simulink model "Ball_and_Plate_MicroLabBox"  (R2019b)
settings: Solver=ode1  StartTime=0.0  StopTime=Inf  FixedStep=0.001  RelTol=1e-3
PostLoadFcn:
  | , if any(exist('dsrtsu_mdlpostloadfcn', 'file') ~= 0), dsrtsu_mdlpostloadfcn('Execute', bdroot); end,
InitFcn:
  | , if any(exist('rtifpga_mdlclblib', 'file') ~= 0), rtifpga_mdlclblib('Init', bdroot); end,
undefined symbols (not defined in the file or in its folder): denc_mi, denco12_dis_des, denF, g, K, Kcam_x, Kcam_y, numc_mi, numco12_dis_des, numF, Ts_Outer
libraries: rtiemclib x6, rti1202lib_dac_class1 x3, rtiethernetlib x3, simulink x1
(part 2 of 2)

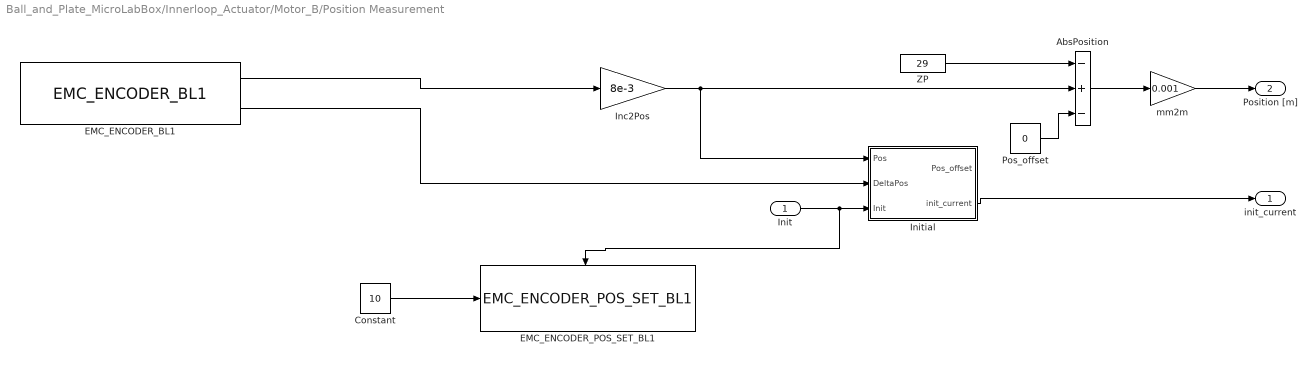
== system Ball_and_Plate_MicroLabBox/Innerloop_Actuator/Motor_B/Position Measurement ==
  Init : Inport
  AbsPosition : Sum  Inputs=-+-  SaturateOnIntegerOverflow=on
  Constant : Constant  Value=10
  EMC_ENCODER_BL1 : rtiemclib/EMC_ENCODER_BL1  DSProperties=struct('RTI',struct('Version',uint32(2),'BlockType',struct('isSLSource',uint8(1),'isSLSink',uint8(0),'isHWSource',uint8(1),'isHWSink',uint8(0),'isSetup',uint8(0),'isInline',uint8(1),'isNonInline',uint8(0),'isInterrupt',uint8(0),'isChannelwise',uint8(1)),'IOBoardType','DSEMC','UnitType','ENCODER','Identifier','ENCODER','DialogType','ML','BlockSet','RTIEMC','SlaveProcessor','NONE'))  RTIBlockInterface=struct('OutputPortsWidth',int32([1 1 1]),'OutputPortsActive',int32([1 1 0]),'OutputPortsName',{{'Position','Speed',['Index Detected']}},'OutputPortsDataType',{{'SS_DOUBLE','SS_DOUBLE','SS_BOOLEAN'}},'InitLevel',3,'IconTransparency','on','BlockDisplay',{{['EMC Encoder\nUnit: 2\nDIO class: 2\nPort: 1\nChannel: 3'],'center'}},'DialogFcn','rtiemcencodergui','BlockName',struct('Token',{{'EMC_ENCODER_BL1'}}))  RTIBlockParameters=struct('UnitNo',{{2,'OFF',[1 6]}},'DioClassNo',{{2,'OFF',[1 2]}},'PortNo',{{1,'OFF',[1 1]}},'ChannelNo',{{3,'OFF',[1 11]}},'HwSignalPin',{{['DIO1 ch1'],'OFF',[]}},'HwRefPin',{{'GND','OFF',[]}},'EnablePosMeasurement',{{1,'OFF',[0 1]}},'IndexSetMode',{{1,'OFF',[1 3]}},'EnableMinSpeed',{{0,'OFF',[0 1]}},'NumOfLines',{{'1024','OFF',[1 2097152]}},'InitAngleValue',{{'60','OFF',[0 359.99999]}},'IndexAngleValue',{{'0','OFF',[0 359.99999]}},'MinSpeedAngleValue',{{'45','OFF',[0.05 10000]}},'MinPosValue',{{'0','OFF',[-2097152 2097150.75]}},'MaxPosValue',{{'10000','OFF',[-2097151 2097151.75]}},'InitPosValue',{{'0','OFF',[-2097152 2097151.75]}},'IndexPosValue',{{'7500','OFF',[-2097152 2097151.75]}},'MinSpeedPosValue',{{'100','OFF',[1 1000000]}},'IndexGateMode',{{0,'OFF',[0 1]}},'EnableNoiseFilter',{{0,'OFF',[0 1]}},'FilterInterval',{{'0','OFF',[0 0.01]}},'IndexDetectedOutPortMode',{{0,'OFF',[0 1]}},'BuildCheckAngleMeasurement',{{0,'OFF',[0 1]}},'BuildCheckAngleIndexMode',{{0,'OFF',[0 1]}},'BuildCheckPosIndexMode',{{0,'OFF',[0 1]}},'BuildCheckAngleMinSpeed',{{0,'OFF',[0 1]}},'BuildCheckPosMinSpeed',{{0,'OFF',[0 1]}},'TLCFileName',{{'rtiemcencoder','OFF',[]}})  RTISFcnParameters=struct('UnitNo','int32','DioClassNo','int32','PortNo','int32','ChannelNo','int32','EnablePosMeasurement','int32','IndexSetMode','int32','IndexDetectedOutPortMode','int32','EnableMinSpeed','int32','NumOfLines','uint32','InitAngleValue','double','IndexAngleValue','double','MinSpeedAngleValue','double','MinPosValue','double','MaxPosValue','double','InitPosValue','double','IndexPosValue','double','MinSpeedPosValue','double','IndexGateMode','int32','EnableNoiseFilter','int32','FilterInterval','double','TLCFileName','char')  RTIBlockParaDefault=struct('UnitNo',1,'DioClassNo',1,'PortNo',1,'ChannelNo',1,'HwSignalPin',['DIO1 ch1'],'HwRefPin','GND','EnablePosMeasurement',0,'IndexSetMode',1,'EnableMinSpeed',0,'NumOfLines',1024,'InitAngleValue',60,'IndexAngleValue',0,'MinSpeedAngleValue',45,'MinPosValue',0,'MaxPosValue',1023.75,'InitPosValue',0,'IndexPosValue',0,'MinSpeedPosValue',100,'IndexGateMode',0,'EnableNoiseFilter',0,'FilterInterval',0,'IndexDetectedOutPortMode',0,'BuildCheckAngleMeasurement',1,'BuildCheckAngleIndexMode',0,'BuildCheckPosIndexMode',0,'BuildCheckAngleMinSpeed',0,'BuildCheckPosMinSpeed',0,'TLCFileName','rtiemcencoder')
      settings: SourceProductName=dSPACE RTI Electric Motor Control Blockset
  EMC_ENCODER_POS_SET_BL1 : rtiemclib/EMC_ENCODER_POS_SET_BL1  DSProperties=struct('RTI',struct('Version',uint32(1),'BlockType',struct('isSLSource',uint8(0),'isSLSink',uint8(1),'isHWSource',uint8(0),'isHWSink',uint8(1),'isSetup',uint8(0),'isInline',uint8(1),'isNonInline',uint8(0),'isInterrupt',uint8(0),'isChannelwise',uint8(1)),'IOBoardType','DSEMC','UnitType','ENCODER','Identifier','ENCODERPOSSET','DialogType','ML','BlockSet','RTIEMC','SlaveProcessor','NONE'))  RTIBlockInterface=struct('InputPortsWidth',int32(1),'InputPortsActive',1,'InputPortsDataType',{{'SS_DOUBLE'}},'InputPortsName',{{'Position'}},'TriggerPort',{{'rising'}},'InitLevel',3,'IconTransparency','on','BlockDisplay',{{['EMC Encoder Position Set\nUnit: 2\nDIO class: 2\nPort: 1\nChannel: 3'],'center'}},'DialogFcn','rtiemcencoderpossetgui','BlockName',struct('Token',{{'EMC_ENCODER_POS_SET_BL1'}}))  RTIBlockParameters=struct('EncoderIdIndex',{{3,'OFF',[1 4]}},'UnitNo',{{2,'OFF',[]}},'DioClassNo',{{2,'OFF',[]}},'PortNo',{{1,'OFF',[]}},'ChannelNo',{{3,'OFF',[]}},'EnablePosMeasurement',{{1,'OFF',[]}},'NumOfLines',{{1024,'OFF',[]}},'TLCFileName',{{'rtiemcencoderposset','OFF',[]}})  RTISFcnParameters=struct('EncoderIdIndex','int32','UnitNo','int32','DioClassNo','int32','PortNo','int32','ChannelNo','int32','EnablePosMeasurement','int32','NumOfLines','int32','TLCFileName','char')  RTIBlockParaDefault=struct('EncoderIdIndex',1,'UnitNo',-1,'DioClassNo',-1,'PortNo',-1,'ChannelNo',-1,'EnablePosMeasurement',0,'NumOfLines',1024,'TLCFileName','rtiemcencoderposset')
      settings: SourceProductName=dSPACE RTI Electric Motor Control Blockset
  Inc2Pos : Gain  Gain=8e-3  SaturateOnIntegerOverflow=on  OutDataTypeStr=Inherit: Same as input  ParamDataTypeStr=Inherit: Same as input
  Initial : Subsystem
  Pos_offset : Constant  Value=0
  ZP : Constant  Value=29
  mm2m : Gain  Gain=0.001
  init_current : Outport  VectorParamsAs1DForOutWhenUnconnected=off
  Position [m] : Outport  Port=2  VectorParamsAs1DForOutWhenUnconnected=off
  wires:
  AbsPosition/1 -> mm2m/1
  Inc2Pos/1 -> Initial/1(Pos), AbsPosition/2
  Initial/2(init_current) -> init_current/1
  mm2m/1 -> Position [m]/1
  EMC_ENCODER_BL1/2 -> Initial/2(DeltaPos)
  ZP/1 -> AbsPosition/1
  Init/1 -> EMC_ENCODER_POS_SET_BL1/Trigger, Initial/3(Init)
  Constant/1 -> EMC_ENCODER_POS_SET_BL1/1
  Pos_offset/1 -> AbsPosition/3
  EMC_ENCODER_BL1/1 -> Inc2Pos/1

== system Ball_and_Plate_MicroLabBox/Innerloop_Actuator/Motor_C/Outputs to Amplifier ==
  Motor current [A] : Inport
  Current2V : Gain  Gain=10/3  SaturateOnIntegerOverflow=on  OutDataTypeStr=Inherit: Same as input  ParamDataTypeStr=Inherit: Same as input
  DAC_CLASS1_BL1 : rti1202lib_dac_class1/DAC_CLASS1_BL1  DSProperties=struct('RTI',struct('Version',uint32(2),'BlockType',struct('isSLSource',uint8(0),'isSLSink',uint8(1),'isHWSource',uint8(0),'isHWSink',uint8(1),'isSetup',uint8(0),'isInline',uint8(1),'isNonInline',uint8(0),'isInterrupt',uint8(0),'isChannelwise',uint8(1)),'IOBoardType',{{'DS120X','STD','DACC1'}},'UnitType','DAC','Identifier','DAC','DialogType','ML','BlockSet','NONE','SlaveProcessor','NONE'))  RTIBlockInterface=struct('InputPortsActive',1,'InputPortsWidth',int32(1),'InputPortsDataType',{{'SS_DOUBLE'}},'InputPortsName',{{['DAC 3']}},'DialogFcn','rti120xstddacc1dacgui','InitLevel',3,'IconTransparency','on','BlockDisplay',{{['DAC CL1\nChannel: 3'],'center'}},'BlockName',struct('Token',{{'DAC_CLASS1_BL1'}}))  RTIBlockParameters=struct('ChannelNo',{{3,'OFF',[]}},'ChannelNumOf',{{1,'OFF',[]}},'InitialValue1',{{'0','OFF',[-10 10]}},'InitialValue2',{{'0','OFF',[-10 10]}},'InitialValue3',{{'0','OFF',[-10 10]}},'InitialValue4',{{'0','OFF',[-10 10]}},'InitialValue5',{{'0','OFF',[-10 10]}},'InitialValue6',{{'0','OFF',[-10 10]}},'InitialValue7',{{'0','OFF',[-10 10]}},'InitialValue8',{{'0','OFF',[-10 10]}},'InitialValue9',{{'0','OFF',[-10 10]}},'InitialValue10',{{'0','OFF',[-10 10]}},'InitialValue11',{{'0','OFF',[-10 10]}},'InitialValue12',{{'0','OFF',[-10 10]}},'InitialValue13',{{'0','OFF',[-10 10]}},'InitialValue14',{{'0','OFF',[-10 10]}},'InitialValue15',{{'0','OFF',[-10 10]}},'InitialValue16',{{'0','OFF',[-10 10]}},'OutputMode',{{ones(1,16),'OFF',[1 2]}},'TermValue1',{{'0','OFF',[-10 10]}},'TermValue2',{{'0','OFF',[-10 10]}},'TermValue3',{{'0','OFF',[-10 10]}},'TermValue4',{{'0','OFF',[-10 10]}},'TermValue5',{{'0','OFF',[-10 10]}},'TermValue6',{{'0','OFF',[-10 10]}},'TermValue7',{{'0','OFF',[-10 10]}},'TermValue8',{{'0','OFF',[-10 10]}},'TermValue9',{{'0','OFF',[-10 10]}},'TermValue10',{{'0','OFF',[-10 10]}},'TermValue11',{{'0','OFF',[-10 10]}},'TermValue12',{{'0','OFF',[-10 10]}},'TermValue13',{{'0','OFF',[-10 10]}},'TermValue14',{{'0','OFF',[-10 10]}},'TermValue15',{{'0','OFF',[-10 10]}},'TermValue16',{{'0','OFF',[-10 10]}},'EnableTermMode',{{0,'OFF',[0 1]}},'TLCFileName',{{'rti120xdac_c1_dac','OFF',[]}},'InitialValueBuildCheck1',{{0,'OFF',[]}},'InitialValueBuildCheck2',{{0,'OFF',[]}},'InitialValueBuildCheck3',{{1,'OFF',[]}},'InitialValueBuildCheck4',{{0,'OFF',[]}},'InitialValueBuildCheck5',{{0,'OFF',[]}},'InitialValueBuildCheck6',{{0,'OFF',[]}},'InitialValueBuildCheck7',{{0,'OFF',[]}},'InitialValueBuildCheck8',{{0,'OFF',[]}},'InitialValueBuildCheck9',{{0,'OFF',[]}},'InitialValueBuildCheck10',{{0,'OFF',[]}},'InitialValueBuildCheck11',{{0,'OFF',[]}},'InitialValueBuildCheck12',{{0,'OFF',[]}},'InitialValueBuildCheck13',{{0,'OFF',[]}},'InitialValueBuildCheck14',{{0,'OFF',[]}},'InitialValueBuildCheck15',{{0,'OFF',[]}},'InitialValueBuildCheck16',{{0,'OFF',[]}},'TermValueBuildCheck1',{{0,'OFF',[]}},'TermValueBuildCheck2',{{0,'OFF',[]}},'TermValueBuildCheck3',{{0,'OFF',[]}},'TermValueBuildCheck4',{{0,'OFF',[]}},'TermValueBuildCheck5',{{0,'OFF',[]}},'TermValueBuildCheck6',{{0,'OFF',[]}},'TermValueBuildCheck7',{{0,'OFF',[]}},'TermValueBuildCheck8',{{0,'OFF',[]}},'TermValueBuildCheck9',{{0,'OFF',[]}},'TermValueBuildCheck10',{{0,'OFF',[]}},'TermValueBuildCheck11',{{0,'OFF',[]}},'TermValueBuildCheck12',{{0,'OFF',[]}},'TermValueBuildCheck13',{{0,'OFF',[]}},'TermValueBuildCheck14',{{0,'OFF',[]}},'TermValueBuildCheck15',{{0,'OFF',[]}},'TermValueBuildCheck16',{{0,'OFF',[]}})  RTISFcnParameters=struct('ChannelNo','int16','ChannelNumOf','int16','InitialValue1','double','InitialValue2','double','InitialValue3','double','InitialValue4','double','InitialValue5','double','InitialValue6','double','InitialValue7','double','InitialValue8','double','InitialValue9','double','InitialValue10','double','InitialValue11','double','InitialValue12','double','InitialValue13','double','InitialValue14','double','InitialValue15','double','InitialValue16','double','OutputMode','int16','TermValue1','double','TermValue2','double','TermValue3','double','TermValue4','double','TermValue5','double','TermValue6','double','TermValue7','double','TermValue8','double','TermValue9','double','TermValue10','double','TermValue11','double','TermValue12','double','TermValue13','double','TermValue14','double','TermValue15','double','TermValue16','double','EnableTermMode','int16','TLCFileName','char')  RTIBlockParaDefault=struct('ChannelNo',1,'ChannelNumOf',1,'InitialValue1',0,'InitialValue2',0,'InitialValue3',0,'InitialValue4',0,'InitialValue5',0,'InitialValue6',0,'InitialValue7',0,'InitialValue8',0,'InitialValue9',0,'InitialValue10',0,'InitialValue11',0,'InitialValue12',0,'InitialValue13',0,'InitialValue14',0,'InitialValue15',0,'InitialValue16',0,'OutputMode',ones(1,16),'TermValue1',0,'TermValue2',0,'TermValue3',0,'TermValue4',0,'TermValue5',0,'TermValue6',0,'TermValue7',0,'TermValue8',0,'TermValue9',0,'TermValue10',0,'TermValue11',0,'TermValue12',0,'TermValue13',0,'TermValue14',0,'TermValue15',0,'TermValue16',0,'EnableTermMode',0,'TLCFileName','rti120xdac_c1_dac','InitialValueBuildCheck1',0,'InitialValueBuildCheck2',0,'InitialValueBuildCheck3',0,'InitialValueBuildCheck4',0,'InitialValueBuildCheck5',0,'InitialValueBuildCheck6',0,'InitialValueBuildCheck7',0,'InitialValueBuildCheck8',0,'InitialValueBuildCheck9',0,'InitialValueBuildCheck10',0,'InitialValueBuildCheck11',0,'InitialValueBuildCheck12',0,'InitialValueBuildCheck13',0,'InitialValueBuildCheck14',0,'InitialValueBuildCheck15',0,'InitialValueBuildCheck16',0,'TermValueBuildCheck1',0,'TermValueBuildCheck2',0,'TermValueBuildCheck3',0,'TermValueBuildCheck4',0,'TermValueBuildCheck5',0,'TermValueBuildCheck6',0,'TermValueBuildCheck7',0,'TermValueBuildCheck8',0,'TermValueBuildCheck9',0,'TermValueBuildCheck10',0,'TermValueBuildCheck11',0,'TermValueBuildCheck12',0,'TermValueBuildCheck13',0,'TermValueBuildCheck14',0,'TermValueBuildCheck15',0,'TermValueBuildCheck16',0)
  DSPscale : Gain  Gain=1/10  SaturateOnIntegerOverflow=on  OutDataTypeStr=Inherit: Same as input  ParamDataTypeStr=Inherit: Same as input
  Saturation : Saturate  UpperLimit=3  LowerLimit=-3
  wires:
  Saturation/1 -> Current2V/1
  Current2V/1 -> DSPscale/1
  Motor current [A]/1 -> Saturation/1
  DSPscale/1 -> DAC_CLASS1_BL1/1

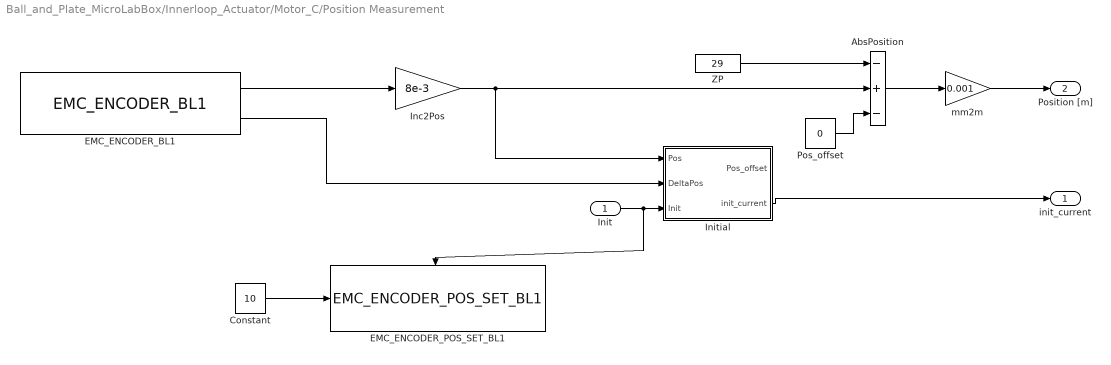
== system Ball_and_Plate_MicroLabBox/Innerloop_Actuator/Motor_C/Position Measurement ==
  Init : Inport
  AbsPosition : Sum  Inputs=-+-  SaturateOnIntegerOverflow=on
  Constant : Constant  Value=10
  EMC_ENCODER_BL1 : rtiemclib/EMC_ENCODER_BL1  DSProperties=struct('RTI',struct('Version',uint32(2),'BlockType',struct('isSLSource',uint8(1),'isSLSink',uint8(0),'isHWSource',uint8(1),'isHWSink',uint8(0),'isSetup',uint8(0),'isInline',uint8(1),'isNonInline',uint8(0),'isInterrupt',uint8(0),'isChannelwise',uint8(1)),'IOBoardType','DSEMC','UnitType','ENCODER','Identifier','ENCODER','DialogType','ML','BlockSet','RTIEMC','SlaveProcessor','NONE'))  RTIBlockInterface=struct('OutputPortsWidth',int32([1 1 1]),'OutputPortsActive',int32([1 1 0]),'OutputPortsName',{{'Position','Speed',['Index Detected']}},'OutputPortsDataType',{{'SS_DOUBLE','SS_DOUBLE','SS_BOOLEAN'}},'InitLevel',3,'IconTransparency','on','BlockDisplay',{{['EMC Encoder\nUnit: 3\nDIO class: 2\nPort: 1\nChannel: 5'],'center'}},'DialogFcn','rtiemcencodergui','BlockName',struct('Token',{{'EMC_ENCODER_BL1'}}))  RTIBlockParameters=struct('UnitNo',{{3,'OFF',[1 6]}},'DioClassNo',{{2,'OFF',[1 2]}},'PortNo',{{1,'OFF',[1 1]}},'ChannelNo',{{5,'OFF',[1 11]}},'HwSignalPin',{{['DIO1 ch1'],'OFF',[]}},'HwRefPin',{{'GND','OFF',[]}},'EnablePosMeasurement',{{1,'OFF',[0 1]}},'IndexSetMode',{{1,'OFF',[1 3]}},'EnableMinSpeed',{{0,'OFF',[0 1]}},'NumOfLines',{{'1024','OFF',[1 2097152]}},'InitAngleValue',{{'60','OFF',[0 359.99999]}},'IndexAngleValue',{{'0','OFF',[0 359.99999]}},'MinSpeedAngleValue',{{'45','OFF',[0.05 10000]}},'MinPosValue',{{'0','OFF',[-2097152 2097150.75]}},'MaxPosValue',{{'10000','OFF',[-2097151 2097151.75]}},'InitPosValue',{{'0','OFF',[-2097152 2097151.75]}},'IndexPosValue',{{'0','OFF',[-2097152 2097151.75]}},'MinSpeedPosValue',{{'100','OFF',[1 1000000]}},'IndexGateMode',{{0,'OFF',[0 1]}},'EnableNoiseFilter',{{0,'OFF',[0 1]}},'FilterInterval',{{'0','OFF',[0 0.01]}},'IndexDetectedOutPortMode',{{0,'OFF',[0 1]}},'BuildCheckAngleMeasurement',{{0,'OFF',[0 1]}},'BuildCheckAngleIndexMode',{{0,'OFF',[0 1]}},'BuildCheckPosIndexMode',{{0,'OFF',[0 1]}},'BuildCheckAngleMinSpeed',{{0,'OFF',[0 1]}},'BuildCheckPosMinSpeed',{{0,'OFF',[0 1]}},'TLCFileName',{{'rtiemcencoder','OFF',[]}})  RTISFcnParameters=struct('UnitNo','int32','DioClassNo','int32','PortNo','int32','ChannelNo','int32','EnablePosMeasurement','int32','IndexSetMode','int32','IndexDetectedOutPortMode','int32','EnableMinSpeed','int32','NumOfLines','uint32','InitAngleValue','double','IndexAngleValue','double','MinSpeedAngleValue','double','MinPosValue','double','MaxPosValue','double','InitPosValue','double','IndexPosValue','double','MinSpeedPosValue','double','IndexGateMode','int32','EnableNoiseFilter','int32','FilterInterval','double','TLCFileName','char')  RTIBlockParaDefault=struct('UnitNo',1,'DioClassNo',1,'PortNo',1,'ChannelNo',1,'HwSignalPin',['DIO1 ch1'],'HwRefPin','GND','EnablePosMeasurement',0,'IndexSetMode',1,'EnableMinSpeed',0,'NumOfLines',1024,'InitAngleValue',60,'IndexAngleValue',0,'MinSpeedAngleValue',45,'MinPosValue',0,'MaxPosValue',1023.75,'InitPosValue',0,'IndexPosValue',0,'MinSpeedPosValue',100,'IndexGateMode',0,'EnableNoiseFilter',0,'FilterInterval',0,'IndexDetectedOutPortMode',0,'BuildCheckAngleMeasurement',1,'BuildCheckAngleIndexMode',0,'BuildCheckPosIndexMode',0,'BuildCheckAngleMinSpeed',0,'BuildCheckPosMinSpeed',0,'TLCFileName','rtiemcencoder')
      settings: SourceProductName=dSPACE RTI Electric Motor Control Blockset
  EMC_ENCODER_POS_SET_BL1 : rtiemclib/EMC_ENCODER_POS_SET_BL1  DSProperties=struct('RTI',struct('Version',uint32(1),'BlockType',struct('isSLSource',uint8(0),'isSLSink',uint8(1),'isHWSource',uint8(0),'isHWSink',uint8(1),'isSetup',uint8(0),'isInline',uint8(1),'isNonInline',uint8(0),'isInterrupt',uint8(0),'isChannelwise',uint8(1)),'IOBoardType','DSEMC','UnitType','ENCODER','Identifier','ENCODERPOSSET','DialogType','ML','BlockSet','RTIEMC','SlaveProcessor','NONE'))  RTIBlockInterface=struct('InputPortsWidth',int32(1),'InputPortsActive',1,'InputPortsDataType',{{'SS_DOUBLE'}},'InputPortsName',{{'Position'}},'TriggerPort',{{'rising'}},'InitLevel',3,'IconTransparency','on','BlockDisplay',{{['EMC Encoder Position Set\nUnit: 3\nDIO class: 2\nPort: 1\nChannel: 5'],'center'}},'DialogFcn','rtiemcencoderpossetgui','BlockName',struct('Token',{{'EMC_ENCODER_POS_SET_BL1'}}))  RTIBlockParameters=struct('EncoderIdIndex',{{4,'OFF',[1 4]}},'UnitNo',{{3,'OFF',[]}},'DioClassNo',{{2,'OFF',[]}},'PortNo',{{1,'OFF',[]}},'ChannelNo',{{5,'OFF',[]}},'EnablePosMeasurement',{{1,'OFF',[]}},'NumOfLines',{{1024,'OFF',[]}},'TLCFileName',{{'rtiemcencoderposset','OFF',[]}})  RTISFcnParameters=struct('EncoderIdIndex','int32','UnitNo','int32','DioClassNo','int32','PortNo','int32','ChannelNo','int32','EnablePosMeasurement','int32','NumOfLines','int32','TLCFileName','char')  RTIBlockParaDefault=struct('EncoderIdIndex',1,'UnitNo',-1,'DioClassNo',-1,'PortNo',-1,'ChannelNo',-1,'EnablePosMeasurement',0,'NumOfLines',1024,'TLCFileName','rtiemcencoderposset')
      settings: SourceProductName=dSPACE RTI Electric Motor Control Blockset
  Inc2Pos : Gain  Gain=8e-3  SaturateOnIntegerOverflow=on  OutDataTypeStr=Inherit: Same as input  ParamDataTypeStr=Inherit: Same as input
  Initial : Subsystem
  Pos_offset : Constant  Value=0
  ZP : Constant  Value=29
  mm2m : Gain  Gain=0.001
  init_current : Outport  VectorParamsAs1DForOutWhenUnconnected=off
  Position [m] : Outport  Port=2  VectorParamsAs1DForOutWhenUnconnected=off
  wires:
  AbsPosition/1 -> mm2m/1
  Inc2Pos/1 -> Initial/1(Pos), AbsPosition/2
  Initial/2(init_current) -> init_current/1
  mm2m/1 -> Position [m]/1
  EMC_ENCODER_BL1/2 -> Initial/2(DeltaPos)
  ZP/1 -> AbsPosition/1
  Constant/1 -> EMC_ENCODER_POS_SET_BL1/1
  Init/1 -> Initial/3(Init), EMC_ENCODER_POS_SET_BL1/Trigger
  Pos_offset/1 -> AbsPosition/3
  EMC_ENCODER_BL1/1 -> Inc2Pos/1

== system Ball_and_Plate_MicroLabBox/RTI Data/RTI Data Store/RTI Data Store ==
  RTI Data Store : Subsystem  mask(RTI_DATA_STORE){}
      mask help:
      | RTI Data Store Block. This block is used by RTI to store internal model dependent data. Deleting this block will result in data loss.
      |
      | NEVER DELETE, COPY, OR MODIFY THIS BLOCK!
      mask Help:
      | RTI Data Store Block. This block is used by RTI to store internal model dependent data. Deleting this block will result in data loss.
      | 
      | NEVER DELETE, COPY, OR MODIFY THIS BLOCK!
      mask Display: text(0.5, 0.5, ' ', 'HorizontalAlignment', 'center');

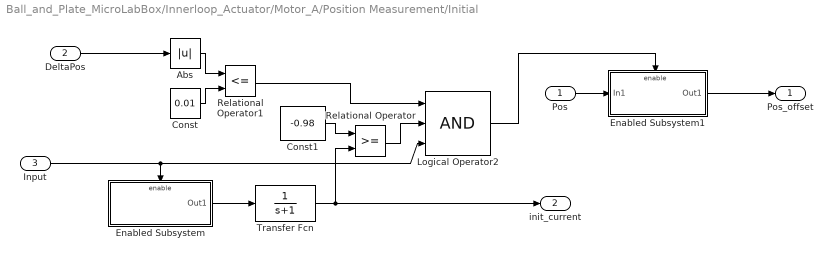
== system Ball_and_Plate_MicroLabBox/Innerloop_Actuator/Motor_A/Position Measurement/Initial ==
  Pos : Inport
  DeltaPos : Inport  Port=2
  Input : Inport  Port=3
  Abs : Abs  SaturateOnIntegerOverflow=on
  Const : Constant  Value=0.01
  Const1 : Constant  Value=-0.98
  Enabled Subsystem : Subsystem  TreatAsAtomicUnit=on
  Enabled Subsystem1 : Subsystem  TreatAsAtomicUnit=on
  Logical Operator2 : Logic  Inputs=3  AllPortsSameDT=off
  Relational Operator : RelationalOperator  RndMeth=Nearest
  Relational Operator1 : RelationalOperator  Operator=<=  RndMeth=Nearest
  Transfer Fcn : TransferFcn  Denominator=[1 1]
  Pos_offset : Outport  VectorParamsAs1DForOutWhenUnconnected=off
  init_current : Outport  Port=2  VectorParamsAs1DForOutWhenUnconnected=off
  wires:
  Enabled Subsystem/1(Out1) -> Transfer Fcn/1
  Transfer Fcn/1 -> Relational Operator/2, init_current/1
  Input/1 -> Enabled Subsystem/Enable, Logical Operator2/3
  Const1/1 -> Relational Operator/1
  Abs/1 -> Relational Operator1/1
  Const/1 -> Relational Operator1/2
  Relational Operator1/1 -> Logical Operator2/1
  Relational Operator/1 -> Logical Operator2/2
  DeltaPos/1 -> Abs/1
  Logical Operator2/1 -> Enabled Subsystem1/Enable
  Pos/1 -> Enabled Subsystem1/1(In1)
  Enabled Subsystem1/1(Out1) -> Pos_offset/1

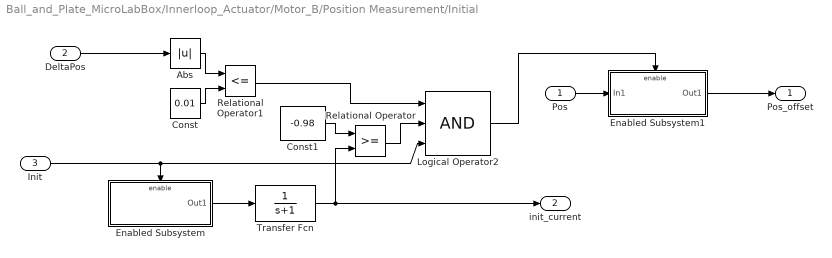
== system Ball_and_Plate_MicroLabBox/Innerloop_Actuator/Motor_B/Position Measurement/Initial ==
  Pos : Inport
  DeltaPos : Inport  Port=2
  Init : Inport  Port=3
  Abs : Abs  SaturateOnIntegerOverflow=on
  Const : Constant  Value=0.01
  Const1 : Constant  Value=-0.98
  Enabled Subsystem : Subsystem  TreatAsAtomicUnit=on
  Enabled Subsystem1 : Subsystem  TreatAsAtomicUnit=on
  Logical Operator2 : Logic  Inputs=3  AllPortsSameDT=off
  Relational Operator : RelationalOperator  RndMeth=Nearest
  Relational Operator1 : RelationalOperator  Operator=<=  RndMeth=Nearest
  Transfer Fcn : TransferFcn  Denominator=[1 1]
  Pos_offset : Outport  VectorParamsAs1DForOutWhenUnconnected=off
  init_current : Outport  Port=2  VectorParamsAs1DForOutWhenUnconnected=off
  wires:
  Enabled Subsystem/1(Out1) -> Transfer Fcn/1
  Transfer Fcn/1 -> Relational Operator/2, init_current/1
  Init/1 -> Enabled Subsystem/Enable, Logical Operator2/3
  Const1/1 -> Relational Operator/1
  Abs/1 -> Relational Operator1/1
  Const/1 -> Relational Operator1/2
  Relational Operator1/1 -> Logical Operator2/1
  Relational Operator/1 -> Logical Operator2/2
  DeltaPos/1 -> Abs/1
  Logical Operator2/1 -> Enabled Subsystem1/Enable
  Pos/1 -> Enabled Subsystem1/1(In1)
  Enabled Subsystem1/1(Out1) -> Pos_offset/1

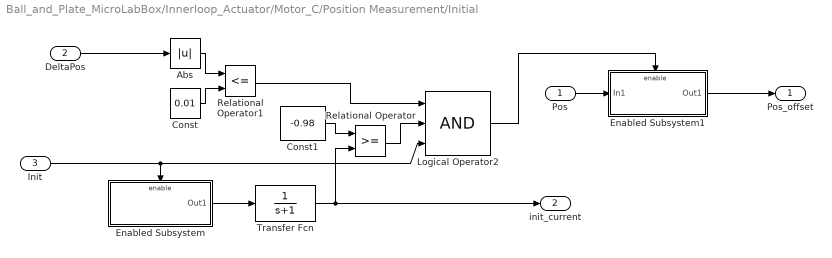
== system Ball_and_Plate_MicroLabBox/Innerloop_Actuator/Motor_C/Position Measurement/Initial ==
  Pos : Inport
  DeltaPos : Inport  Port=2
  Init : Inport  Port=3
  Abs : Abs  SaturateOnIntegerOverflow=on
  Const : Constant  Value=0.01
  Const1 : Constant  Value=-0.98
  Enabled Subsystem : Subsystem  TreatAsAtomicUnit=on
  Enabled Subsystem1 : Subsystem  TreatAsAtomicUnit=on
  Logical Operator2 : Logic  Inputs=3  AllPortsSameDT=off
  Relational Operator : RelationalOperator  RndMeth=Nearest
  Relational Operator1 : RelationalOperator  Operator=<=  RndMeth=Nearest
  Transfer Fcn : TransferFcn  Denominator=[1 1]
  Pos_offset : Outport  VectorParamsAs1DForOutWhenUnconnected=off
  init_current : Outport  Port=2  VectorParamsAs1DForOutWhenUnconnected=off
  wires:
  Enabled Subsystem/1(Out1) -> Transfer Fcn/1
  Transfer Fcn/1 -> Relational Operator/2, init_current/1
  Init/1 -> Enabled Subsystem/Enable, Logical Operator2/3
  Const1/1 -> Relational Operator/1
  Abs/1 -> Relational Operator1/1
  Const/1 -> Relational Operator1/2
  Relational Operator1/1 -> Logical Operator2/1
  Relational Operator/1 -> Logical Operator2/2
  DeltaPos/1 -> Abs/1
  Logical Operator2/1 -> Enabled Subsystem1/Enable
  Pos/1 -> Enabled Subsystem1/1(In1)
  Enabled Subsystem1/1(Out1) -> Pos_offset/1

== system Ball_and_Plate_MicroLabBox/RTI Data/RTI Data Store/RTI Data Store/RTI Data Store ==
  RTI Data Store : Subsystem  mask(RTI_DATA_STORE){}
      mask help:
      | RTI Data Store Block. This block is used by RTI to store internal model dependent data. Deleting this block will result in data loss.
      |
      | NEVER DELETE, COPY, OR MODIFY THIS BLOCK!
      mask Help:
      | RTI Data Store Block. This block is used by RTI to store internal model dependent data. Deleting this block will result in data loss.
      | 
      | NEVER DELETE, COPY, OR MODIFY THIS BLOCK!
      mask Display: text(0.5, 0.5, ' ', 'HorizontalAlignment', 'center');

== system Ball_and_Plate_MicroLabBox/Innerloop_Actuator/Motor_A/Position Measurement/Initial/Enabled Subsystem ==
  Enable : EnablePort  PropagateVarSize=During execution
  Constant : Constant  Value=-1
  Out1 : Outport  OutputWhenDisabled=reset  InitialOutput=[0]  VectorParamsAs1DForOutWhenUnconnected=off
  wires:
  Constant/1 -> Out1/1

== system Ball_and_Plate_MicroLabBox/Innerloop_Actuator/Motor_A/Position Measurement/Initial/Enabled Subsystem1 ==
  In1 : Inport
  Enable : EnablePort  PropagateVarSize=During execution
  Out1 : Outport  InitialOutput=[0]  VectorParamsAs1DForOutWhenUnconnected=off
  wires:
  In1/1 -> Out1/1

== system Ball_and_Plate_MicroLabBox/Innerloop_Actuator/Motor_B/Position Measurement/Initial/Enabled Subsystem ==
  Enable : EnablePort  PropagateVarSize=During execution
  Constant : Constant  Value=-1
  Out1 : Outport  OutputWhenDisabled=reset  InitialOutput=[0]  VectorParamsAs1DForOutWhenUnconnected=off
  wires:
  Constant/1 -> Out1/1

== system Ball_and_Plate_MicroLabBox/Innerloop_Actuator/Motor_B/Position Measurement/Initial/Enabled Subsystem1 ==
  In1 : Inport
  Enable : EnablePort  PropagateVarSize=During execution
  Out1 : Outport  InitialOutput=[0]  VectorParamsAs1DForOutWhenUnconnected=off
  wires:
  In1/1 -> Out1/1

== system Ball_and_Plate_MicroLabBox/Innerloop_Actuator/Motor_C/Position Measurement/Initial/Enabled Subsystem ==
  Enable : EnablePort  PropagateVarSize=During execution
  Constant : Constant  Value=-1
  Out1 : Outport  OutputWhenDisabled=reset  InitialOutput=[0]  VectorParamsAs1DForOutWhenUnconnected=off
  wires:
  Constant/1 -> Out1/1

== system Ball_and_Plate_MicroLabBox/Innerloop_Actuator/Motor_C/Position Measurement/Initial/Enabled Subsystem1 ==
  In1 : Inport
  Enable : EnablePort  PropagateVarSize=During execution
  Out1 : Outport  InitialOutput=[0]  VectorParamsAs1DForOutWhenUnconnected=off
  wires:
  In1/1 -> Out1/1

== system Ball_and_Plate_MicroLabBox/RTI Data/RTI Data Store/RTI Data Store/RTI Data Store/RTI Data Store ==

== matlab function Ball_and_Plate_MicroLabBox/Innerloop_Actuator/MATLAB Function ==
  data: alpha input; beta input; psi input; P_A_ref output; P_B_ref output; P_C_ref output; L_in1 output; L_in2 output; L_in3 output
function [P_A_ref,P_B_ref,P_C_ref,L_in1,L_in2,L_in3] = myfunc(alpha,beta,psi)

%% Rotation matrices

%    Z rotation with angle  psi
RotZ  = [cos(psi) -sin(psi) 0;
         sin(psi)  cos(psi) 0;
          0          0      1]
      
%    Y rotation with angle beta+
RotY  = [cos(beta)       0         sin(beta);
             0           1             0    ;
         -sin(beta)      0        cos(beta)]
    
%    X rotation with angle alpha
RotX  = [1            0                 0    ;
         0        cos(alpha)      -sin(alpha);
         0        sin(alpha)       cos(alpha)]
Rot_BtoP = RotZ*RotY*RotX

%% Specification of the base plate and plate

%Location of motors on the base plate 
r_base = 0.17;               %radii of the base plate (m)
B1     = [r_base; 0; 0]      %position of motor wrt base plate origin
B2     = [-0.5*r_base; (sqrt(3)/2)*r_base; 0]  %120degrees wrt the position of first motor and base plate origin
B3     = [-0.5*r_base; -(sqrt(3)/2)*r_base; 0] %240 degrees wrt first motor and base plate origin

%Location of joints on the plate 
r_plate = 0.17;               %radii of the plate (m)
P1     = [r_plate; 0; 0]      %position of motor wrt base plate origin
P2     = [-0.5*r_plate; (sqrt(3)/2)*r_plate; 0]  %120degrees wrt the position of first motor and base plate origin
P3     = [-0.5*r_plate; -(sqrt(3)/2)*r_plate; 0] %240 degrees wrt first motor and base plate origin

% distance from base plate origin(OXYZ) to plate origin(oxyz)
T = [0; 0; 0.322]                     %30 cm height from (OXYZ) to (oxyz)

%% 
L_in1 = T + (Rot_BtoP*P1)-B1       %change of position of lin motor 1
P_A_ref = sqrt(L_in1(1,1)^2+L_in1(2,1)^2+L_in1(3,1)^2)   %length of L_in1 for passing to motor tf

L_in2 = T + (Rot_BtoP*P2)-B2
P_B_ref = sqrt(L_in2(1,1)^2+L_in2(2,1)^2+L_in2(3,1)^2)

L_in3 = T + (Rot_BtoP*P3)-B3 
P_C_ref = sqrt(L_in3(1,1)^2+L_in3(2,1)^2+L_in3(3,1)^2)
end

== matlab function Ball_and_Plate_MicroLabBox/Innerloop_Actuator/MATLAB Function1 ==
  data: Delta_P_A input; Alpha_angle output; Delta_P_B input; Delta_P_C input; L_in1 input; L_in2 input; L_in3 input; Beta_angle output; Psi_angle output; T_back output
function [Alpha_angle,Beta_angle,Psi_angle,T_back]      = myfunc(Delta_P_A,Delta_P_B,Delta_P_C,L_in1,L_in2,L_in3)



%% Specification of the base plate and plate

%Location of motors on the base plate 
r_base = 0.17;               %radii of the base plate (m)
B1     = [r_base; 0; 0]      %position of motor wrt base plate origin
B2     = [-0.5*r_base; (sqrt(3)/2)*r_base; 0]  %120degrees wrt the position of first motor and base plate origin
B3     = [-0.5*r_base; -(sqrt(3)/2)*r_base; 0] %240 degrees wrt first motor and base plate origin

%Location of joints on the plate 
r_plate = 0.17;               %radii of the plate (m)
P1     = [r_plate; 0; 0];      %position of motor wrt base plate origin
P2     = [-0.5*r_plate; (sqrt(3)/2)*r_plate; 0];  %120degrees wrt the position of first motor and base plate origin
P3     = [-0.5*r_plate; -(sqrt(3)/2)*r_plate; 0]; %240 degrees wrt first motor and base plate origin

% distance from base plate origin(OXYZ) to plate origin(oxyz)
T = [0; 0; 0.322]                     %30 cm height from (OXYZ) to (oxyz)

%actuator plate connections in base frame
% P1b= B1+(L_in1)-T;
% P2b= B2+(L_in2)-T;
% P3b= B3+(L_in3)-T;

P1b= B1+(L_in1*(Delta_P_A))-T;
P2b= B2+(L_in2*(Delta_P_B))-T;
P3b= B3+(L_in3*(Delta_P_C))-T;

%base frame unit vectors
UnitX=[1;0;0];
UnitY=[0;1;0];
UnitZ=[0;0;1];
UnitXp=P1b/sqrt(dot(P1b,P1b));
UnitZp=cross(UnitXp,P3b);
UnitZp=UnitZp/sqrt(dot(UnitZp,UnitZp)); %now length 1
UnitYp=cross(UnitXp,UnitZp);

%this is according to https://en.wikipedia.org/wiki/Euler_angles, Tait-Bryn
%angles

Beta_angle=asin(-UnitXp(3))
Psi_angle=asin(UnitXp(2)/sqrt(1-UnitXp(3)^2))
Alpha_angle=asin(UnitYp(3)/sqrt(1-UnitXp(3)^2))

%Calculating rotation matrix with above angles
RotZ1  = [cos(Psi_angle) -sin(Psi_angle) 0;
         sin(Psi_angle)  cos(Psi_angle) 0;
          0          0      1];
      
%    Y rotation with angle beta
RotY1  = [cos(Beta_angle)       0         sin(Beta_angle);
             0                           1             0    ;
         -sin(Beta_angle)      0        cos(Beta_angle)];
    
%    X rotation with angle alpha
RotX1  = [1            0                                 0    ;
         0        cos(Alpha_angle)      -sin(Alpha_angle);
         0        sin(Alpha_angle)       cos(Alpha_angle)];

% Calculating back the T matrix which was the height between the base plate
% and plate. They must be the same.
Rm_times_P = RotZ1*RotY1*RotX1
T_back = L_in1+B1-(Rm_times_P*P1)

end
